simulink model "lqr_integral_tracking_scheme"  (R2025b)
settings: Solver=VariableStepAuto  StartTime=0.0  StopTime=t_sim  RelTol=1e-3
values from neighbouring files (symbols this model uses):
  Cd = sys_dt.C    [lqr_integral_tracking.m]    (also in lqr_zero_regulation.m)
  Kq = Kaug(1)    [lqr_integral_tracking.m]
  Kx = Kaug(2:n+1)    [lqr_integral_tracking.m]
  Ts = 0.05    [lqr_integral_tracking.m]    (also in lqr_zero_regulation.m)
  x0i = 0    [lqr_integral_tracking.m]
undefined symbols (not defined in the file or in its folder): DiscIntNeverNeededParam
libraries: cstblocks x1
settings Model: Creator=nicol  LastModifiedBy=nicol

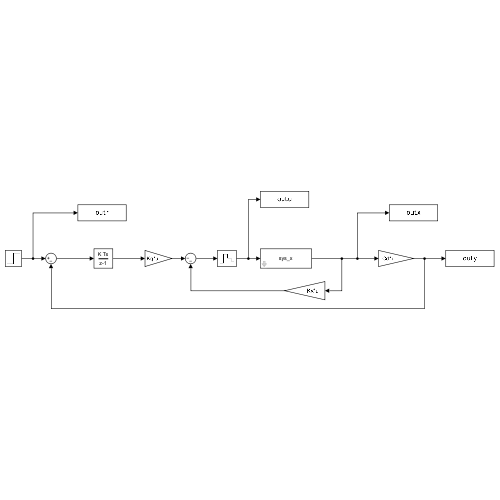
[thumbnail: Simulink's stored preview of the top-level diagram]
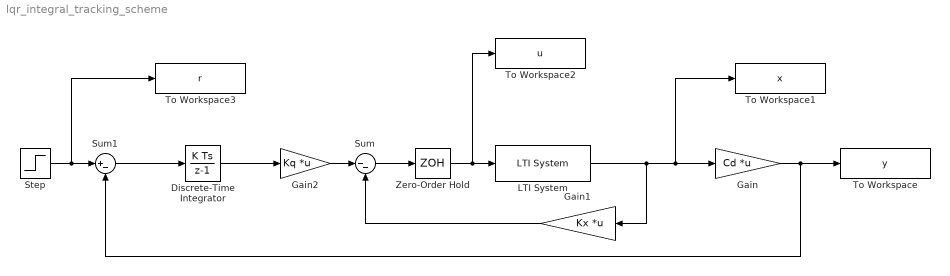
== system lqr_integral_tracking_scheme ==
  Discrete-Time Integrator : DiscreteIntegrator  InitialCondition=x0i  SampleTime=Ts  ICPrevOutput=DiscIntNeverNeededParam  ICPrevScaledInput=DiscIntNeverNeededParam
  Gain : Gain  Gain=Cd  Multiplication=Matrix(K*u)
  Gain1 : Gain  Gain=Kx  Multiplication=Matrix(K*u)
  Gain2 : Gain  Gain=Kq  Multiplication=Matrix(K*u)
  LTI System : cstblocks/LTI System  sys=sys_x  IC=x0  PadeOrder=0
  Step : Step  Time=0  SampleTime=Ts
  Sum : Sum  Inputs=|--
  Sum1 : Sum  Inputs=|+-
  To Workspace : ToWorkspace  VariableName=y  SaveFormat=Timeseries  SampleTime=-1
  To Workspace1 : ToWorkspace  VariableName=x  SaveFormat=Timeseries  SampleTime=-1
  To Workspace2 : ToWorkspace  VariableName=u  SaveFormat=Timeseries  SampleTime=-1
  To Workspace3 : ToWorkspace  VariableName=r  SaveFormat=Timeseries  SampleTime=-1
  Zero-Order Hold : ZeroOrderHold  SampleTime=Ts
  wires:
  Gain1/1 -> Sum/2
  LTI System/1 -> Gain1/1, Gain/1, To Workspace1/1
  Gain/1 -> Sum1/2, To Workspace/1
  Sum/1 -> Zero-Order Hold/1
  Zero-Order Hold/1 -> LTI System/1, To Workspace2/1
  Gain2/1 -> Sum/1
  Discrete-Time Integrator/1 -> Gain2/1
  Sum1/1 -> Discrete-Time Integrator/1
  Step/1 -> To Workspace3/1, Sum1/1
